simulink model "Task26"  (R2025a)
settings: Solver=VariableStepAuto  StartTime=0.0  StopTime=10.0  RelTol=1e-3
settings Model: Creator=LOQ  LastModifiedBy=LOQ

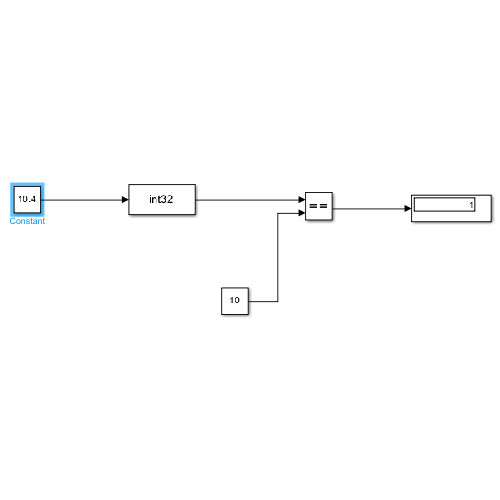
[thumbnail: Simulink's stored preview of the top-level diagram]
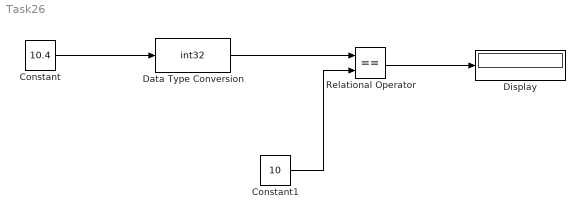
== system Task26 ==
  Constant : Constant  Value=10.4
  Constant1 : Constant  Value=10
  Data Type Conversion : DataTypeConversion  OutDataTypeStr=int32  RndMeth=Round  SaturateOnIntegerOverflow=off
  Display : Display
  Relational Operator : RelationalOperator  Operator===  OutDataTypeStr=boolean  RndMeth=Simplest  InputSameDT=off
  wires:
  Constant/1 -> Data Type Conversion/1
  Data Type Conversion/1 -> Relational Operator/1
  Constant1/1 -> Relational Operator/2
  Relational Operator/1 -> Display/1
